simulink model "simulink_8mars"  (R2024a)
settings: Solver=VariableStepAuto  StartTime=0.0  StopTime=2000  RelTol=1e-3
settings Model: Creator=sabri  LastModifiedBy=MADER143

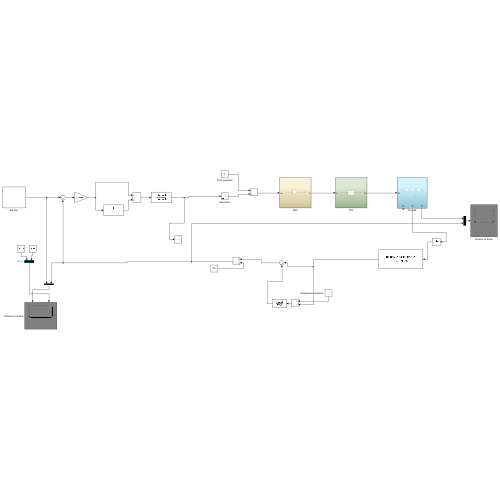
[thumbnail: Simulink's stored preview of the top-level diagram]
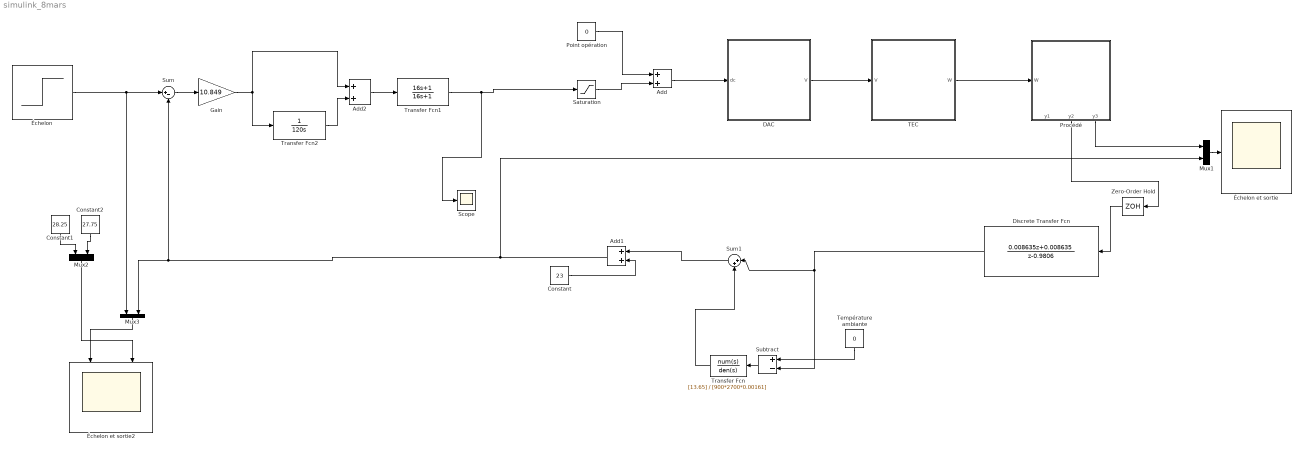
== system simulink_8mars ==
  Add : Sum
  Add1 : Sum
  Add2 : Sum
  Constant : Constant  Value=23
  Constant1 : Constant  Value=28.25
  Constant2 : Constant  Value=27.75
  DAC : Subsystem
  Discrete Transfer Fcn : DiscreteTransferFcn  Numerator=[0.008635 0.008635]  Denominator=[1 -0.9806]
  Gain : Gain  Gain=10.849
  Mux1 : Mux  Inputs=2
  Mux2 : Mux  Inputs=2
  Mux3 : Mux  Inputs=2
  Point opération : Constant  Value=0
  Procédé : Subsystem
      settings: PortSchema="{\"entries\":[{\"content\":{\"sides\":[{\"content\":{\"connectorIds\":[\"In1\"]},\"type\":\"ConnectorPlacement.EquallySpacedRectSide\",\"uuid\":\"20a23230-a41b-4fdf-8ae4-039aa17abee7\"},{\"content\":{\"side\":\"RIGHT\"},\"type\":\"ConnectorPlacement.EquallySpacedRectSide\",\"uuid\":\"82e4e468-e0ad-4c9f-b6ff-cc9c1ee7ea9d\"},{\"content\":{\"side\":\"TOP\"},\"type\":\"ConnectorPlacement.EquallySpacedRectSide\",\"uuid\":\"049bc4af-9a9a-43aa-9803-dca862d69d2b\"},{\"content\":{\"connectorIds\":[\"Out1\",\"Out2\",\"Out3\"],\"side\":\"BOTTOM\"},\"type\":\"ConnectorPlacement.EquallySpacedRectSide\",\"uuid\":\"142d2b37-1c32-477b-9e70-4e4bc8b2913e\"}]},\"type\":\"ConnectorPlacement.EquallySpacedConnector\",\"uuid\":\"a0abf580-2deb-4a1c-9cb8-1272669a26fd\"}],\"packageUris\":[\"http://schema.mathworks.com/mf0/Connector/R2020b\"],\"version\":\"1.0\"}"
  Saturation : Saturate  UpperLimit=255  LowerLimit=-255
  Scope : Scope
  Subtract : Sum  Inputs=+-
  Sum : Sum  Inputs=|+-
  Sum1 : Sum  Inputs=|++
  TEC : Subsystem
  Température ambiante : Constant  Value=0
  Transfer Fcn : TransferFcn  Numerator=[13.65]  Denominator=[900*2700*0.00161]
  Transfer Fcn1 : TransferFcn  Numerator=[16 1]  Denominator=[16 1]
  Transfer Fcn2 : TransferFcn  Denominator=[120 0]
  Zero-Order Hold : ZeroOrderHold  SampleTime=0.5
  Échelon : Step  Time=10  Before=23  After=28  SampleTime=0
  Échelon et sortie : Scope
  Échelon et sortie2 : Scope  NumInputPorts=2
  wires:
  Add/1 -> DAC/1(dc)
  Mux1/1 -> Échelon et sortie/1
  Point opération/1 -> Add/1
  Échelon/1 -> Sum/1, Mux3/1
  Procédé/3(y3) -> Mux1/1
  Procédé/2(y2) -> Zero-Order Hold/1
  Zero-Order Hold/1 -> Discrete Transfer Fcn/1
  Constant/1 -> Add1/2
  Add1/1 -> Mux1/2, Mux3/2, Sum/2
  Sum/1 -> Gain/1
  Gain/1 -> Transfer Fcn2/1, Add2/1
  Transfer Fcn2/1 -> Add2/2
  Add2/1 -> Transfer Fcn1/1
  Saturation/1 -> Add/2
  TEC/1(W) -> Procédé/1(W)
  DAC/1(V) -> TEC/1(V)
  Transfer Fcn1/1 -> Scope/1, Saturation/1
  Subtract/1 -> Transfer Fcn/1
  Transfer Fcn/1 -> Sum1/2
  Discrete Transfer Fcn/1 -> Sum1/1, Subtract/2
  Sum1/1 -> Add1/1
  Température ambiante/1 -> Subtract/1
  Constant1/1 -> Mux2/1
  Constant2/1 -> Mux2/2
  Mux2/1 -> Échelon et sortie2/2
  Mux3/1 -> Échelon et sortie2/1

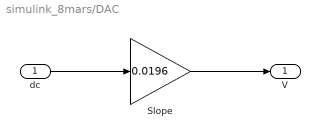
== system simulink_8mars/DAC ==
  dc : Inport
  Slope : Gain  Gain=0.0196
  V : Outport
  wires:
  dc/1 -> Slope/1
  Slope/1 -> V/1

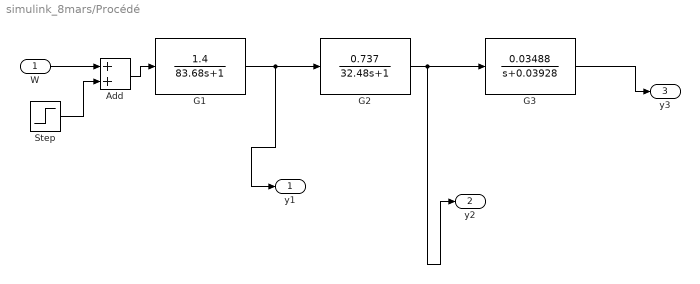
== system simulink_8mars/Procédé ==
  W : Inport
  Add : Sum
  G1 : TransferFcn  Numerator=[1.4]  Denominator=[83.68 1]
  G2 : TransferFcn  Numerator=[0.737]  Denominator=[32.48 1]
  G3 : TransferFcn  Numerator=[0.03488]  Denominator=[1 0.03928]
  Step : Step  Time=60  After=0  SampleTime=0
  y1 : Outport
  y2 : Outport  Port=2
  y3 : Outport  Port=3
  wires:
  G1/1 -> y1/1, G2/1
  Add/1 -> G1/1
  W/1 -> Add/1
  Step/1 -> Add/2
  G2/1 -> G3/1, y2/1
  G3/1 -> y3/1

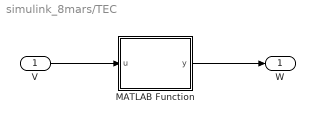
== system simulink_8mars/TEC ==
  V : Inport
  MATLAB Function : MATLAB Function  TreatAsAtomicUnit=on
  W : Outport
  wires:
  V/1 -> MATLAB Function/1(u)
  MATLAB Function/1(y) -> W/1

== matlab function simulink_8mars/TEC/MATLAB Function ==
  data: u input; y output
function y = fcn(u)
y=6.15*u;
